simulink model "ae3e1"  (R2022a)
settings: Solver=FixedStepAuto  StartTime=0.0  StopTime=10.0  FixedStep=0.1  RelTol=1e-3
undefined symbols (not defined in the file): sldvsubsys
libraries: sldvlib x1
settings Model: Creator=attit  LastModifiedBy=attit
settings ConfigComp: DVMode=PropertyProving  DVTestSuiteOptimization=Auto  DVDetectOutOfBounds=on  DVModelReferenceHarness=on  DVHarnessSource=Signal Editor

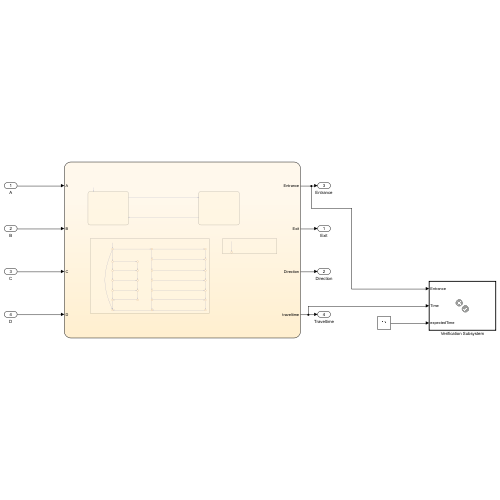
[thumbnail: Simulink's stored preview of the top-level diagram]
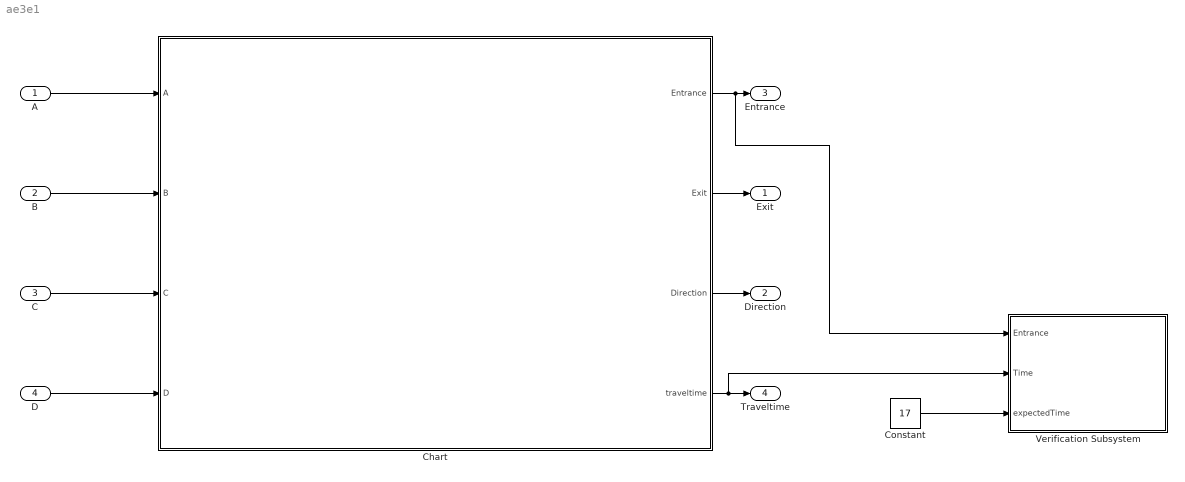
== system ae3e1 ==
  A : Inport  OutDataTypeStr=boolean
  B : Inport  Port=2  OutDataTypeStr=boolean
  C : Inport  Port=3  OutDataTypeStr=boolean
  D : Inport  Port=4  OutDataTypeStr=boolean
  Chart : Stateflow chart  TreatAsAtomicUnit=on
  Constant : Constant  Value=17
  Verification Subsystem : Subsystem  Tag=VerificationSubsystem  DisableCoverage=on  LoadFcn=sldvsubsys('check')  TreatAsAtomicUnit=on  SimViewingDevice=on  mask(VerificationSubsystem){}
      mask init:
      | sldvsubsys('maskInit');
      settings: CopyFcn=sldvsubsys('copy');  OpenFcn=open_system(gcb,'force');
      settings: PreSaveFcn=|
      | set_param(gcb,'SimViewingDevice','on');
      | sldvsubsys('check');
      mask Help: helpview(fullfile(docroot,'toolbox','sldv','sldv.map'),'verificationsubsystem')
      mask Display: image(imread('sldvicon_versubsys.png','BackGroundColor',[1 1 1]),'center');
  Exit : Outport
  Direction : Outport  Port=2
  Entrance : Outport  Port=3
  Traveltime : Outport  Port=4
  wires:
  D/1 -> Chart/4(D)
  C/1 -> Chart/3(C)
  B/1 -> Chart/2(B)
  A/1 -> Chart/1(A)
  Chart/3(Direction) -> Direction/1
  Chart/2(Exit) -> Exit/1
  Chart/4(traveltime) -> Verification Subsystem/2(Time), Traveltime/1
  Chart/1(Entrance) -> Verification Subsystem/1(Entrance), Entrance/1
  Constant/1 -> Verification Subsystem/3(expectedTime)

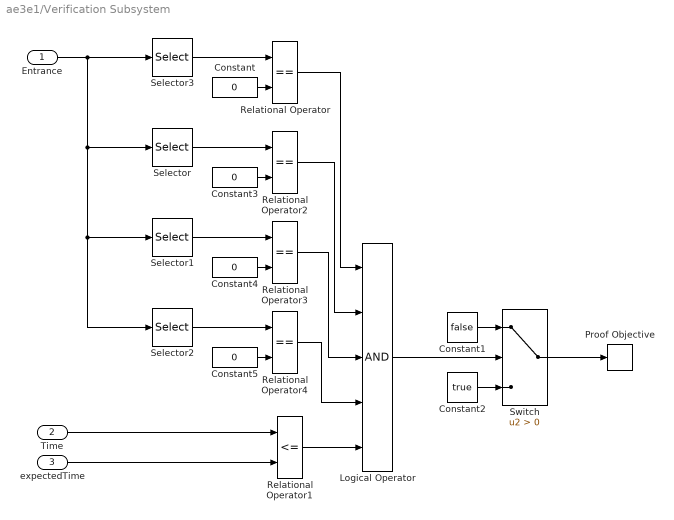
== system ae3e1/Verification Subsystem ==
  Entrance : Inport
  Time : Inport  Port=2
  expectedTime : Inport  Port=3
  Constant{,3..5} (4 alike) : Constant  Value=0  OutDataTypeStr=uint8
  Constant1 : Constant  Value=false
  Constant2 : Constant  Value=true
  Logical Operator : Logic  Inputs=5  AllPortsSameDT=off  OutDataTypeStr=boolean
  Proof Objective : sldvlib/Objectives and Constraints/Proof Objective  enabled=on  customAVTBlockType=Proof Objective  intervals=true  dispValues=on  outEnabled=off  enableStopSim=off
      settings: AttributesFormatString=%<intervals>  SourceProductBaseCode=SL
  Relational Operator{,2..4} (4 alike) : RelationalOperator  Operator===  OutDataTypeStr=boolean  RndMeth=Simplest  InputSameDT=off
  Relational Operator1 : RelationalOperator  Operator=<=  OutDataTypeStr=boolean  RndMeth=Simplest  InputSameDT=off
  Selector : Selector  InputPortWidth=4  IndexOptions=Index vector (dialog)  Indices=2  OutputSizes=1
  Selector1 : Selector  InputPortWidth=4  IndexOptions=Index vector (dialog)  Indices=3  OutputSizes=1
  Selector2 : Selector  InputPortWidth=4  IndexOptions=Index vector (dialog)  Indices=4  OutputSizes=1
  Selector3 : Selector  InputPortWidth=4  IndexOptions=Index vector (dialog)  Indices=1  OutputSizes=1
  Switch : Switch  Criteria=u2 > Threshold  SaturateOnIntegerOverflow=off  InputSameDT=off
  wires:
  Relational Operator2/1 -> Logical Operator/2
  Selector2/1 -> Relational Operator4/1
  Relational Operator/1 -> Logical Operator/1
  Entrance/1 -> Selector2/1, Selector1/1, Selector/1, Selector3/1
  Constant2/1 -> Switch/3
  Selector1/1 -> Relational Operator3/1
  Relational Operator4/1 -> Logical Operator/4
  Constant4/1 -> Relational Operator3/2
  Relational Operator1/1 -> Logical Operator/5
  Switch/1 -> Proof Objective/1
  Constant/1 -> Relational Operator/2
  Logical Operator/1 -> Switch/2
  Relational Operator3/1 -> Logical Operator/3
  Selector/1 -> Relational Operator2/1
  Constant3/1 -> Relational Operator2/2
  Selector3/1 -> Relational Operator/1
  Constant5/1 -> Relational Operator4/2
  Constant1/1 -> Switch/1
  Time/1 -> Relational Operator1/1
  expectedTime/1 -> Relational Operator1/2

== stateflow chart ae3e1/Chart ==
  state Entrance
    en:
    Direction = true ;
  state Exit
    en:
    Direction = false ;
  state check = Crossing(Direction1,A1,B1,C1,D1,Entrance1,Exit1) [function]
    (default) -> (junction 8) : {inputs = [A1 B1 C1 D1];...
        | check = false;}
    (junction 8) -> (junction 25) [order 1] : [Direction1==1&&length(find(inputs))==2]
    (junction 25) -> (junction 31) [order 1] : [A1==true && B1 == true && Entrance1(1)==true&&Entrance1(2)==true]
    (junction 8) -> (junction 29) [order 3]
    (junction 8) -> (junction 27) [order 2] : [Direction1==0 &&length(find(inputs))==1]
    (junction 25) -> (junction 33) [order 2]
    (junction 31) -> (junction 35)
    (junction 33) -> (junction 35) [order 1] : [A1==true && C1 == true && Entrance1(1)==true&&Entrance1(3)==true]
    (junction 33) -> (junction 39) [order 2]
    (junction 35) -> (junction 41)
    (junction 27) -> (junction 66) [order 1] : [A1==true && Exit1(1)==true]
    (junction 27) -> (junction 74) [order 2]
    (junction 66) -> (junction 68)
    (junction 74) -> (junction 68) [order 1] : [B1==true && Exit1(2)==true]
    (junction 39) -> (junction 41) [order 1] : [A1==true && D1 == true && Entrance1(1)==true&&Entrance1(4)==true]
    (junction 74) -> (junction 77) [order 2]
    (junction 68) -> (junction 70)
    (junction 39) -> (junction 44) [order 2]
    (junction 41) -> (junction 46)
    (junction 77) -> (junction 70) [order 1] : [C1==true && Exit1(3)==true]
    (junction 44) -> (junction 46) [order 1] : [B1==true && C1 == true && Entrance1(2)==true&&Entrance1(3)==true]
    (junction 77) -> (junction 80) [order 2]
    (junction 70) -> (junction 72)
    (junction 44) -> (junction 49) [order 2]
    (junction 46) -> (junction 51)
    (junction 80) -> (junction 72) [order 1] : [D1==true && Exit1(4)==true]
    (junction 49) -> (junction 51) [order 1] : [B1==true && D1 == true && Entrance1(2)==true&&Entrance1(4)==true]
    (junction 80) -> (junction 85) [order 2]
    (junction 72) -> (junction 83)
    (junction 49) -> (junction 54) [order 2]
    (junction 51) -> (junction 56)
    (junction 83) -> (junction 85) : {check = true;}
    (junction 54) -> (junction 56) [order 1] : [C1==true && D1 == true && Entrance1(3)==true&&Entrance1(4)==true]
    (junction 85) -> (junction 29)
    (junction 54) -> (junction 59) [order 2]
    (junction 56) -> (junction 61)
    (junction 59) -> (junction 29)
    (junction 61) -> (junction 59) : {check = true;}
  state longestTime = timing(timevalues1,A1,B1,C1,D1) [function]
    (default) -> (junction 113) : {k = find([A1,B1,C1,D1],1,'last');
        | longestTime=timevalues1(k(1));}
  (default) -> Entrance
  Entrance -> Exit : [Crossing(Direction,A,B,C,D,Entrance,Exit)]
      | {traveltime = traveltime + timing(timevalues,A,B,C,D) ;
      | Entrance(find([A B C D],1,'first'))= false;
      | Entrance(find([A B C D],1,'last'))= false;}
  Exit -> Entrance : [Crossing(Direction,A,B,C,D,Entrance,Exit)]
      | {traveltime = timing(timevalues,A,B,C,D)+ traveltime;
      | Exit(find([A B C D],1))=false;}
  data: Direction1 function_input; check function_output; A1 function_input; B1 function_input; C1 function_input; D1 function_input; Entrance1 function_input; Exit1 function_input; timevalues1 function_input; A1 function_input; B1 function_input; C1 function_input; D1 function_input; longestTime function_output; A input boolean; B input boolean; C input boolean; D input boolean; inputs local boolean size=[1 4] =[false false false false]; Entrance output boolean size=[1 4] =[true true true true]; Exit output boolean size=[1 4] =[false false false false]; Direction output boolean; traveltime output uint8 =uint8(0); timevalues local uint8 =uint8([1 2 5 10])
